simulink model "model"  (R2022b)
settings: Solver=VariableStepAuto  StartTime=0.0  StopTime=10.0  RelTol=1e-3
settings Model: Creator=antek  LastModifiedBy=antek

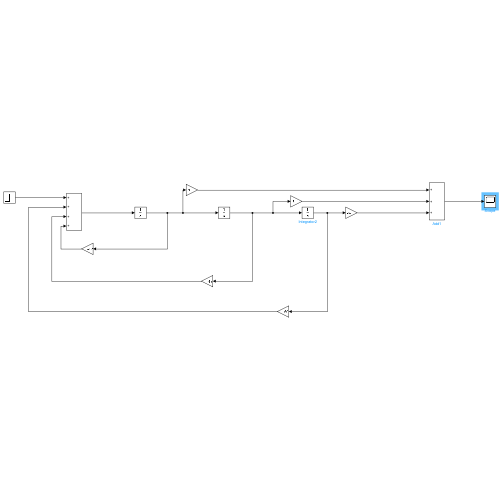
[thumbnail: Simulink's stored preview of the top-level diagram]
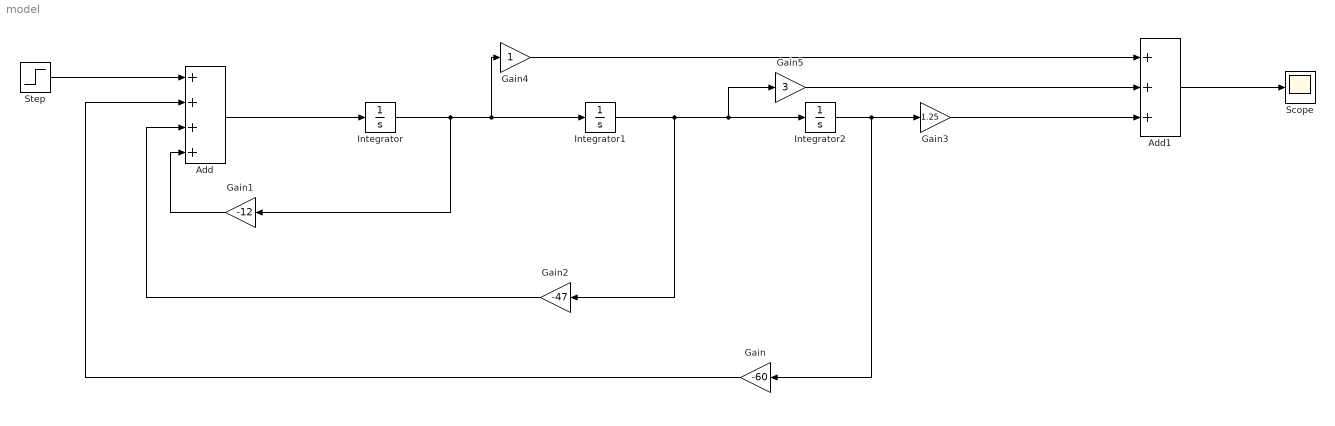
== system model ==
  Add : Sum  Inputs=++++
  Add1 : Sum  Inputs=+++
  Gain : Gain  Gain=-60
  Gain1 : Gain  Gain=-12
  Gain2 : Gain  Gain=-47
  Gain3 : Gain  Gain=1.25
  Gain4 : Gain
  Gain5 : Gain  Gain=3
  Integrator : Integrator
  Integrator1 : Integrator
  Integrator2 : Integrator
  Scope : Scope
  Step : Step  SampleTime=0
  wires:
  Integrator/1 -> Gain1/1, Gain4/1, Integrator1/1
  Integrator1/1 -> Gain2/1, Gain5/1, Integrator2/1
  Step/1 -> Add/1
  Add/1 -> Integrator/1
  Gain1/1 -> Add/4
  Gain2/1 -> Add/3
  Integrator2/1 -> Gain/1, Gain3/1
  Gain3/1 -> Add1/3
  Gain/1 -> Add/2
  Gain5/1 -> Add1/2
  Gain4/1 -> Add1/1
  Add1/1 -> Scope/1
